simulink model "TRASL_S"  (R2024b)
settings: Solver=VariableStepAuto  StartTime=0.0  StopTime=5  MaxStep=0.01  RelTol=1e-3
InitFcn:
  | m1 = 290;
  | m2 = 59;
  | b1 = 1000;
  | k1 = 16182;
  | k2 = 19000;
  | f = 0;

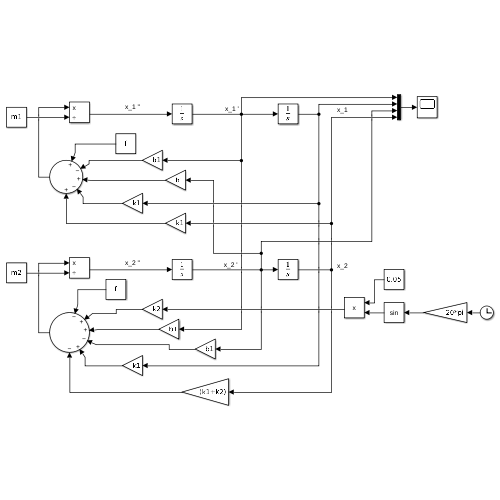
[thumbnail: Simulink's stored preview of the top-level diagram]
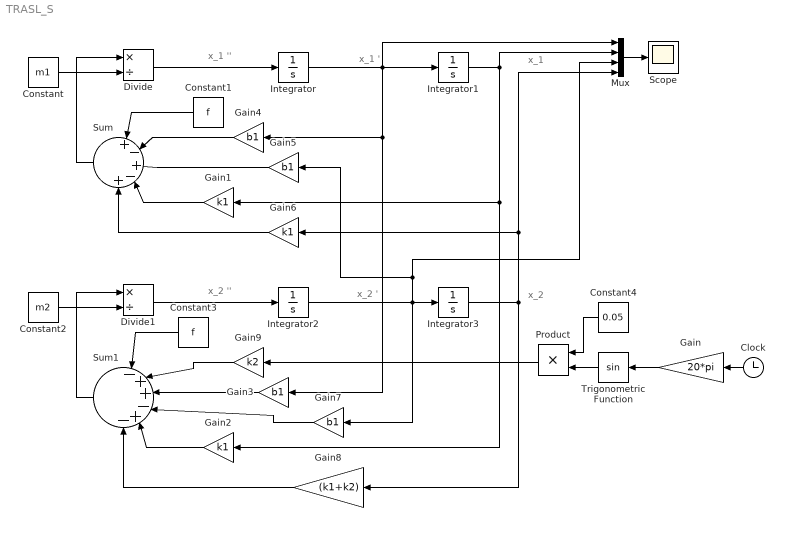
== system TRASL_S ==
  note: x_1 '
  note: x_1
  note: x_1 ''
  note: x_2 '
  note: x_2
  note: x_2 ''
  Clock : Clock
  Constant : Constant  Value=m1
  Constant1 : Constant  Value=f
  Constant2 : Constant  Value=m2
  Constant3 : Constant  Value=f
  Constant4 : Constant  Value=0.05
  Divide : Product  Inputs=*/
  Divide1 : Product  Inputs=*/
  Gain : Gain  Gain=20*pi
  Gain1 : Gain  Gain=k1
  Gain2 : Gain  Gain=k1
  Gain{3..5,7} (4 alike) : Gain  Gain=b1
  Gain6 : Gain  Gain=k1
  Gain8 : Gain  Gain=(k1+k2)
  Gain9 : Gain  Gain=k2
  Integrator{,1..3} (4 alike) : Integrator
  Mux : Mux
  Product : Product
  Scope : Scope
  Sum : Sum  Inputs=|+|-|+|-|+
  Sum1 : Sum  Inputs=|-|+|+|-|+|-
  Trigonometric Function : Trigonometry
  wires:
  Mux/1 -> Scope/1
  Integrator/1 -> Gain3/1, Gain4/1, Mux/1, Integrator1/1
  Divide/1 -> Integrator/1
  Constant/1 -> Divide/2
  Constant1/1 -> Sum/1
  Sum/1 -> Divide/1
  Gain4/1 -> Sum/2
  Gain1/1 -> Sum/4
  Constant3/1 -> Sum1/1
  Integrator3/1 -> Gain8/1, Mux/4, Gain6/1
  Divide1/1 -> Integrator2/1
  Integrator2/1 -> Gain7/1, Mux/3, Gain5/1, Integrator3/1
  Sum1/1 -> Divide1/1
  Constant2/1 -> Divide1/2
  Gain5/1 -> Sum/3
  Gain6/1 -> Sum/5
  Gain3/1 -> Sum1/3
  Gain7/1 -> Sum1/4
  Gain2/1 -> Sum1/5
  Integrator1/1 -> Gain2/1, Gain1/1, Mux/2
  Gain8/1 -> Sum1/6
  Clock/1 -> Gain/1
  Product/1 -> Gain9/1
  Gain9/1 -> Sum1/2
  Trigonometric Function/1 -> Product/2
  Gain/1 -> Trigonometric Function/1
  Constant4/1 -> Product/1
